simulink model "ex2"  (Simulink 7.9)
settings: Solver=ode45  StartTime=0.0  StopTime=10.0  RelTol=1e-3
settings Model: Creator=Daniel  LastModifiedBy=Daniel

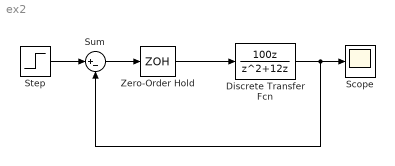
== system ex2 ==
  Discrete Transfer Fcn : DiscreteTransferFcn  Numerator=[0 100 0]  Denominator=[1 12 0]
  Scope : Scope
  Step : Step  SampleTime=0
  Sum : Sum  Inputs=|+-
  Zero-Order Hold : ZeroOrderHold
  wires:
  Zero-Order Hold/1 -> Discrete Transfer Fcn/1
  Discrete Transfer Fcn/1 -> Scope/1, Sum/2
  Step/1 -> Sum/1
  Sum/1 -> Zero-Order Hold/1
